simulink model "PhyMod_PwrEntryCalc"  (R2016b)
settings: configuration reference "CodeGenConfigSet" (kept outside this file)
values from neighbouring files (symbols this model uses):
  CALORIFIC_VALUE = fi(42.5,)    [init_PhyMod_PwrEntryCalc.m]
  Epm_numCyl_C = uint8(4)    [init_PhyMod_PwrEntryCalc.m]
  PhyMod_pwrEGLos_MAP = Calibration.Parameter    [init_PhyMod_PwrEntryCalc.m]
  PhyMod_pwrEGLos_MAPX = Calibration.Parameter    [init_PhyMod_PwrEntryCalc.m]
  PhyMod_pwrEGLos_MAPY = Calibration.Parameter    [init_PhyMod_PwrEntryCalc.m]
  VEHMOT_PI = fi(3.1416,)    [init_PhyMod_PwrEntryCalc.m]
settings Model: Creator=Administrator  LastModifiedBy=wangrui
settings ConfigSetRef: SourceLocation=Base Workspace

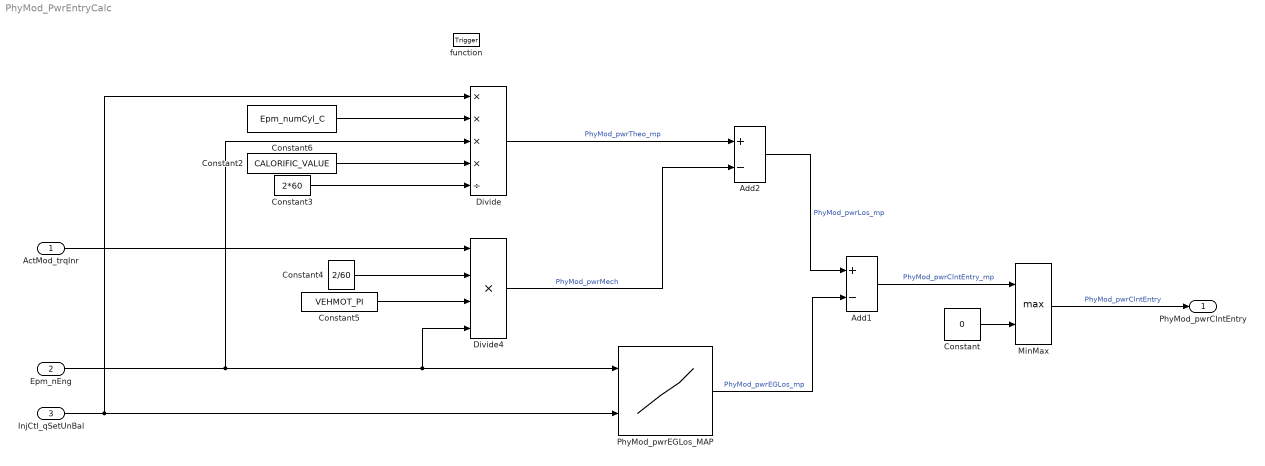
== system PhyMod_PwrEntryCalc ==
  ActMod_trqInr : Inport  Tag=Nm  Description=Current, back-calculated inner engine torque  OutMin=-3276.8  OutMax=3276.7  OutDataTypeStr=Trq_Nm
  Epm_nEng : Inport  Tag=rpm  Description=Engine speed  Port=2  OutMin=-12000  OutMax=12000  OutDataTypeStr=EngSpeed_rpm
  InjCtl_qSetUnBal : Inport  Tag=mg/hub  Description=Current injection quantity  Port=3  OutMin=-319  OutMax=319  OutDataTypeStr=FuelMass_mg_hub
  function : TriggerPort  TriggerType=function-call  VariantControl=Variant
  Add1 : Sum  Inputs=+-  OutDataTypeStr=Inherit: Inherit via back propagation  InputSameDT=on
  Add2 : Sum  Inputs=+-  OutDataTypeStr=Inherit: Inherit via back propagation  InputSameDT=on
  Constant : Constant  Value=0  OutDataTypeStr=Inherit: Inherit via back propagation
  Constant2 : Constant  Value=CALORIFIC_VALUE  OutDataTypeStr=fixdt(0,8,2)
  Constant3 : Constant  Value=2*60  OutDataTypeStr=uint8
  Constant4 : Constant  Value=2/60  OutDataTypeStr=fixdt(0,16,14)
  Constant5 : Constant  Value=VEHMOT_PI  OutDataTypeStr=fixdt(0,16,10)
  Constant6 : Constant  Value=Epm_numCyl_C
  Divide : Product  Inputs=****/  OutDataTypeStr=Pwrl
  Divide4 : Product  Inputs=****  OutDataTypeStr=Pwrl
  MinMax : MinMax  Function=max  Inputs=2  InputSameDT=on
  PhyMod_pwrEGLos_MAP : Lookup_n-D  BreakpointsForDimension1=PhyMod_pwrEGLos_MAPY  BreakpointsForDimension2=PhyMod_pwrEGLos_MAPX  IndexSearchMethod=Linear search  BeginIndexSearchUsingPreviousIndexResult=on  Table=PhyMod_pwrEGLos_MAP  ExtrapMethod=Clip  UseLastTableValue=on  InternalRulePriority=Speed  OutDataTypeStr=Inherit: Inherit via back propagation  SaturateOnIntegerOverflow=on
  PhyMod_pwrClntEntry : Outport  Tag=W  Description=Engine power entry into the coolant water  OutMin=-214748364  OutMax=214748364  OutDataTypeStr=Pwrl
  wires:
  Constant/1 -> MinMax/2
  InjCtl_qSetUnBal/1 -> PhyMod_pwrEGLos_MAP/2, Divide/1
  Add2/1 -> Add1/1  "PhyMod_pwrLos_mp"
  Divide/1 -> Add2/1  "PhyMod_pwrTheo_mp"
  Add1/1 -> MinMax/1  "PhyMod_pwrClntEntry_mp"
  Constant4/1 -> Divide4/2
  Constant2/1 -> Divide/4
  Epm_nEng/1 -> Divide/3, Divide4/4, PhyMod_pwrEGLos_MAP/1
  PhyMod_pwrEGLos_MAP/1 -> Add1/2  "PhyMod_pwrEGLos_mp"
  MinMax/1 -> PhyMod_pwrClntEntry/1  "PhyMod_pwrClntEntry"
  ActMod_trqInr/1 -> Divide4/1
  Divide4/1 -> Add2/2  "PhyMod_pwrMech"
  Constant3/1 -> Divide/5
  Constant5/1 -> Divide4/3
  Constant6/1 -> Divide/2
